simulink model "House_OneNodeModel_mdl"  (R2016b)
settings: Solver=ode45  StartTime=0.0  StopTime=2*24*3600  MaxStep=100  RelTol=1e-3  EnableMultiTasking=on
libraries: carnot x3
settings Model: Creator=drhf  LastModifiedBy=drhf
settings DataIOCC: SaveFormat=Array  SignalLoggingSaveFormat=ModelDataLogs
settings OptimizationCC: ExpressionDepthLimit=2147483647  LifeSpan=inf
settings DebuggingCC: UnderspecifiedInitializationDetection=Classic  MergeDetectMultiDrivingBlocksExec=none  SolverPrmCheckMsg=warning  FcnCallInpInsideContextMsg=warning  StateNameClashWarn=warning  SFUnexpectedBacktrackingDiag=warning  SFNoUnconditionalDefaultTransitionDiag=warning  SFExecutionAtInitializationDiag=none
settings HardwareCC: ProdBitPerPointer=32  ProdBitPerSizeT=32  ProdBitPerPtrDiffT=32  ProdLargestAtomicFloat=None  ProdIntDivRoundTo=Undefined  ProdEndianess=Unspecified  ProdWordSize=32  ProdHWDeviceType=32-bit Generic
settings ModelReferenceCC: PropagateSignalLabelsOutOfModel=off
settings GRTTargetCC: TargetLangStandard=C89/C90 (ANSI)  GeneratePreprocessorConditionals=Disable all  CombineOutputUpdateFcns=off  GRTInterface=on
settings ConfigComp: CovMetricSettings=dw  CovHtmlReporting=on  CovSaveCumulativeToWorkspaceVar=on  CovSaveSingleToWorkspaceVar=on  CovExternalEMLEnable=off

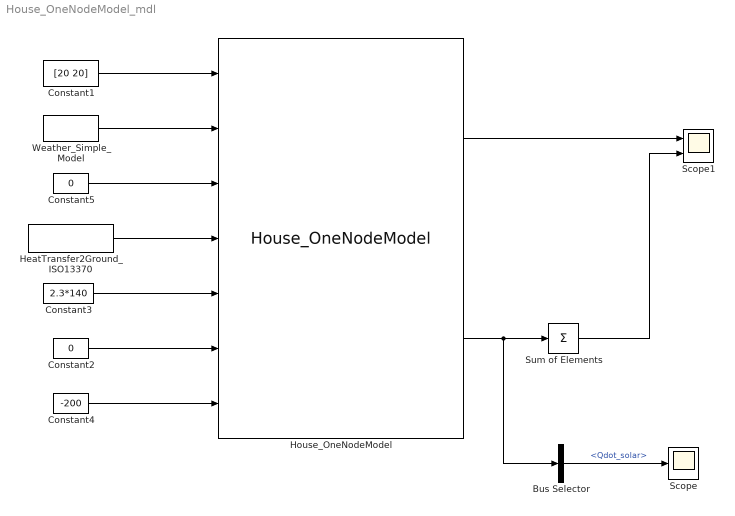
== system House_OneNodeModel_mdl ==
  Bus Selector : BusSelector  OutputSignals=Qdot_solar
  Constant1 : Constant  Value=[20 20]
  Constant2 : Constant  Value=0
  Constant3 : Constant  Value=2.3*140
  Constant4 : Constant  Value=-200
  Constant5 : Constant  Value=0
  HeatTransfer2Ground_ISO13370 : carnot/Load/Houses/heat_transfer/HeatTransfer2Ground_ISO13370  wallsize=[7 10]  gammat=0  Tmeaninside=23.8  deltathetai=3.8  Tmeanoutside=11  deltathetae=9.3  tshift=319*3600  dwall=0.4  cond_ground=2.0  cp_ground=800  rho_ground=2500  rtot=1./0.183
  House_OneNodeModel : carnot/Basic/Thermal_Models/House_OneNodeModel  A=140  UAout=0.197*(54.6+26.4)+0.286*((45.7+56.0)*2 -(12+4+3+4))  UAin=[1.5 1.5]  capa=0.5e6  tini=20  dtroom=inf  AziWin=[0 90 -180 -90]  Awin=[12 4 3 4]  Uwin="[1    1   1    1]*1.5"  Gwin="[1    1   1    1]*0.622*(1-0.15)"
  Scope : Scope
  Scope1 : Scope  NumInputPorts=2
  Sum of Elements : Sum  Inputs=+
  Weather_Simple_Model : carnot/Weather/Weather_Simple_Model  lat=60  Ibn=900  Idg=100  tamb=5  deltaTsky=-1  rh=50  precip="10e-3/24/3600           % 10 mm in 24 h"  cloud=0.125  p=1013e2  vw=1  wdir=270
  wires:
  Weather_Simple_Model/1 -> House_OneNodeModel/2
  House_OneNodeModel/1 -> Scope1/1
  Constant1/1 -> House_OneNodeModel/1
  HeatTransfer2Ground_ISO13370/1 -> House_OneNodeModel/4
  Constant2/1 -> House_OneNodeModel/6
  Constant5/1 -> House_OneNodeModel/3
  Constant4/1 -> House_OneNodeModel/7
  House_OneNodeModel/2 -> Bus Selector/1, Sum of Elements/1
  Sum of Elements/1 -> Scope1/2
  Constant3/1 -> House_OneNodeModel/5
  Bus Selector/1 -> Scope/1  "<Qdot_solar>"
